simulink model "motor_cc_controlled_velocity_US"  (R2015b)
settings: Solver=ode15s  StartTime=0.0  StopTime=5  FixedStep=0.1  RelTol=1e-3
undefined symbols (not defined in the file): f, J, Ke, Km, L, R
settings Model: Creator=Ivan  LastModifiedBy=Ivan
settings DataIOCC: SaveFormat=Array  SignalLoggingSaveFormat=ModelDataLogs
settings OptimizationCC: ExpressionDepthLimit=2147483647  InitFltsAndDblsToZero=on
settings DebuggingCC: SaveWithParameterizedLinksMsg=none  UnderspecifiedInitializationDetection=Classic  MergeDetectMultiDrivingBlocksExec=none  SignalResolutionControl=TryResolveAllWithWarning  SolverPrmCheckMsg=warning  MultiTaskDSMMsg=warning  MultiTaskCondExecSysMsg=none  FcnCallInpInsideContextMsg=UseLocalSettings  StateNameClashWarn=warning
settings HardwareCC: ProdBitPerPointer=32  ProdLargestAtomicFloat=None  ProdIntDivRoundTo=Undefined  ProdEndianess=Unspecified  ProdWordSize=32  ProdHWDeviceType=32-bit Generic
settings GRTTargetCC: TargetFcnLib=ansi_tfl_tmw.mat  GeneratePreprocessorConditionals=Disable all  CombineOutputUpdateFcns=off  GRTInterface=on
settings ConfigComp: CovModelRefEnable=Off

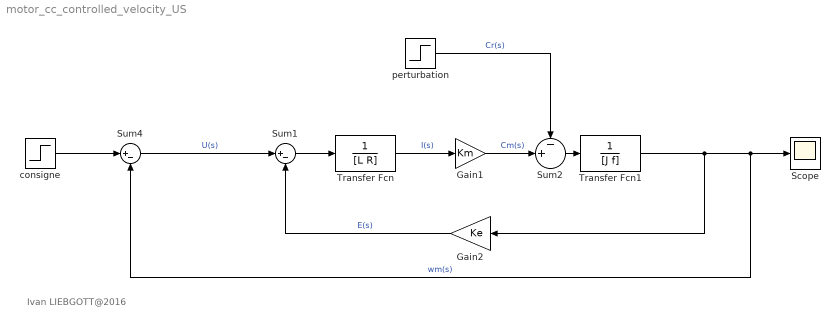
== system motor_cc_controlled_velocity_US ==
  note: Ivan LIEBGOTT@2016
  Gain1 : Gain  Gain=Km
  Gain2 : Gain  Gain=Ke
  Scope : Scope
  Sum1 : Sum  Inputs=|+-
  Sum2 : Sum  Inputs=-+|
  Sum4 : Sum  Inputs=|+-
  Transfer Fcn : TransferFcn  Denominator=[L R]
  Transfer Fcn1 : TransferFcn  Denominator=[J f]
  consigne : Step  Time=0  SampleTime=0
  perturbation : Step  Time=0  After=0  SampleTime=0
  wires:
  Sum1/1 -> Transfer Fcn/1
  Gain2/1 -> Sum1/2  "E(s)"
  Transfer Fcn/1 -> Gain1/1  "I(s)"
  Sum2/1 -> Transfer Fcn1/1
  perturbation/1 -> Sum2/1  "Cr(s)"
  Transfer Fcn1/1 -> Scope/1, Sum4/2, Gain2/1  "wm(s)"
  Sum4/1 -> Sum1/1  "U(s)"
  consigne/1 -> Sum4/1
  Gain1/1 -> Sum2/2  "Cm(s)"
